simulink model "car_control_byKeyboard"  (R2023a)
settings: Solver=VariableStepAuto  StartTime=0.0  StopTime=inf  RelTol=1e-3
settings Model: Creator=15113  LastModifiedBy=15113

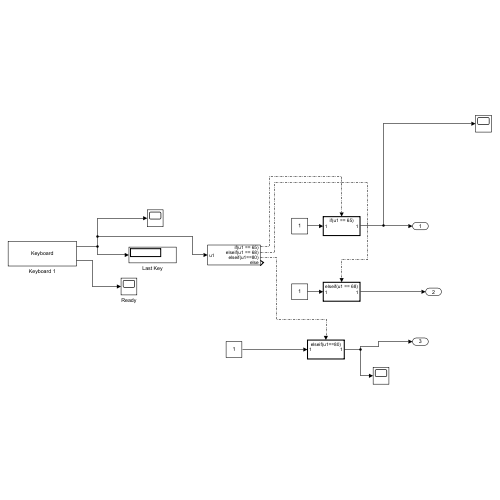
[thumbnail: Simulink's stored preview of the top-level diagram]
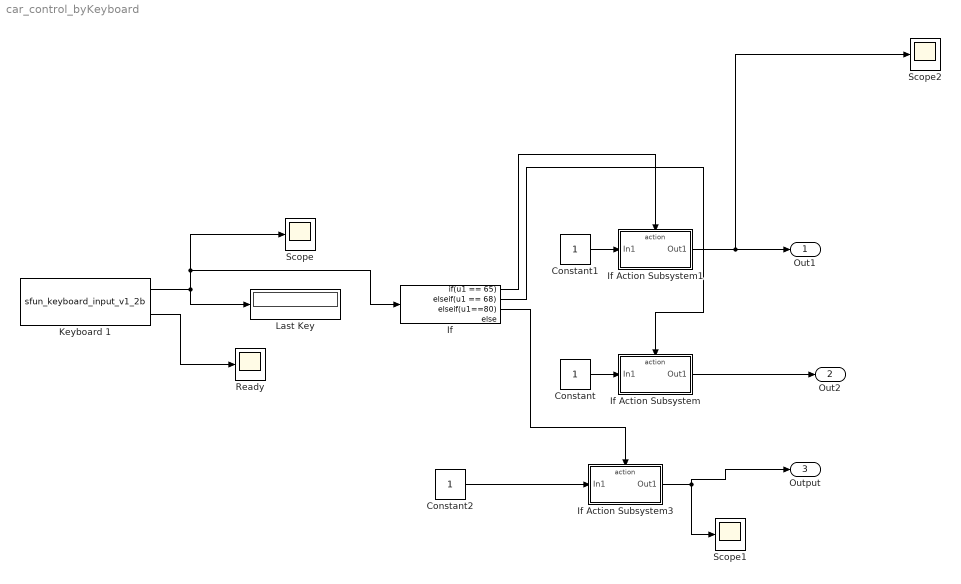
== system car_control_byKeyboard ==
  Constant : Constant
  Constant1 : Constant
  Constant2 : Constant
  If : If  IfExpression=u1 == 65  ElseIfExpressions=u1 == 68,u1==80
  If Action Subsystem : Subsystem  TreatAsAtomicUnit=on
  If Action Subsystem1 : Subsystem  TreatAsAtomicUnit=on
  If Action Subsystem3 : Subsystem  TreatAsAtomicUnit=on
  Keyboard 1 : M-S-Function  FunctionName=sfun_keyboard_input_v1_2b  mask(Keyboard Input){}
      mask help: Keyboard Input
      mask Display: fprintf('Keyboard');
  Last Key : Display
  Ready : Scope
  Scope : Scope
  Scope1 : Scope
  Scope2 : Scope
  Out1 : Outport
  Out2 : Outport  Port=2
  Output : Outport  Port=3
  wires:
  Keyboard 1/1 -> If/1, Scope/1, Last Key/1
  Keyboard 1/2 -> Ready/1
  If Action Subsystem1/1(Out1) -> Scope2/1, Out1/1
  If/2 -> If Action Subsystem/Action
  If Action Subsystem/1(Out1) -> Out2/1
  Constant/1 -> If Action Subsystem/1(In1)
  Constant1/1 -> If Action Subsystem1/1(In1)
  Constant2/1 -> If Action Subsystem3/1(In1)
  If Action Subsystem3/1(Out1) -> Output/1, Scope1/1
  If/1 -> If Action Subsystem1/Action
  If/3 -> If Action Subsystem3/Action

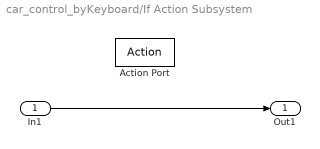
== system car_control_byKeyboard/If Action Subsystem ==
  In1 : Inport
  Action Port : ActionPort  ActionPortLabel=elseif(u1 == 68)
  Out1 : Outport
  wires:
  In1/1 -> Out1/1

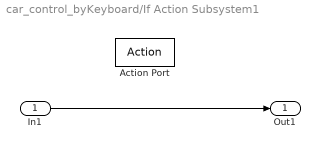
== system car_control_byKeyboard/If Action Subsystem1 ==
  In1 : Inport
  Action Port : ActionPort  ActionPortLabel=if(u1 == 65)
  Out1 : Outport
  wires:
  In1/1 -> Out1/1

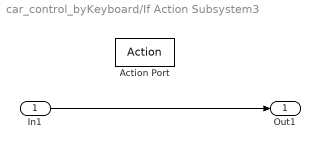
== system car_control_byKeyboard/If Action Subsystem3 ==
  In1 : Inport
  Action Port : ActionPort  ActionPortLabel=elseif(u1==80)
  Out1 : Outport
  wires:
  In1/1 -> Out1/1
